simulink model "jMPC_simulinkNL"  (R2022b)
settings: Solver=ode23s  StartTime=0.0  StopTime=simopts.simulink.Tfinal  FixedStep=simopts.Ts  RelTol=1e-3  EnableMultiTasking=on
undefined symbols (not defined in the file): SIMJMPC, simopts
libraries: jMPClib x2, simulink x1
settings Model: Creator=Jonathan  LastModifiedBy=Jonathan Currie
settings SolverCC: AlgebraicLoopSolver=TrustRegion
settings DataIOCC: LimitDataPoints=on  SaveFormat=Array  SignalLoggingSaveFormat=ModelDataLogs  ReturnWorkspaceOutputs=off
settings OptimizationCC: ExpressionDepthLimit=2147483647  LifeSpan=inf
settings DebuggingCC: UnderspecifiedInitializationDetection=Classic  MergeDetectMultiDrivingBlocksExec=none  SolverPrmCheckMsg=warning  FcnCallInpInsideContextMsg=warning  UnconnectedInputMsg=warning  UnconnectedOutputMsg=warning  UnconnectedLineMsg=warning  StateNameClashWarn=warning  SFUnexpectedBacktrackingDiag=warning  SFNoUnconditionalDefaultTransitionDiag=warning  SFExecutionAtInitializationDiag=none  SFMachineParentedDataDiag=warning  ArithmeticOperatorsInVariantConditions=warning
settings HardwareCC: ProdBitPerPointer=32  ProdBitPerSizeT=32  ProdBitPerPtrDiffT=32  ProdLargestAtomicFloat=None  ProdIntDivRoundTo=Undefined  ProdEndianess=Unspecified  ProdWordSize=32  ProdHWDeviceType=32-bit Generic
settings ModelReferenceCC: PropagateSignalLabelsOutOfModel=off
settings SFSimCC: SimUseLocalCustomCode=off  CustomCodeUndefinedFunction=UseInterfaceOnly
settings RTWCC: RTWUseLocalCustomCode=off
settings CodeAppCC: StateflowObjectComments=on
settings GRTTargetCC: TargetLangStandard=C89/C90 (ANSI)  CombineOutputUpdateFcns=off  GRTInterface=on
settings ConfigComp: CovMetricSettings=dw  CovSaveCumulativeToWorkspaceVar=on  CovSaveSingleToWorkspaceVar=on  CovExternalEMLEnable=off

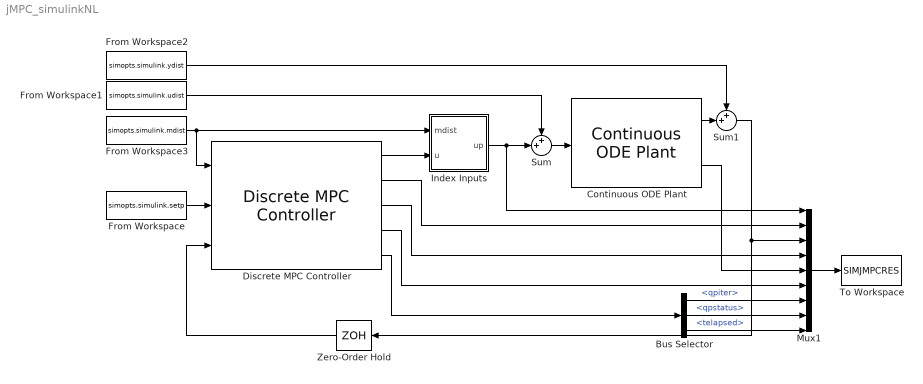
== system jMPC_simulinkNL ==
  Bus Selector : BusSelector  OutputSignals=qpiter,qpstatus,telapsed
  Continuous ODE Plant : jMPClib/MPC Blocks/Continuous ODE Plant  jNLObj=SIMJMPCPlant
      settings: SourceProductName=JMPC Toolbox
  Discrete MPC Controller : jMPClib/MPC Blocks/Discrete MPC Controller  SIMJMPC=SIMJMPC
      settings: SourceProductName=JMPC Toolbox
  From Workspace : FromWorkspace  VariableName=simopts.simulink.setp  SampleTime=simopts.Ts
  From Workspace1 : FromWorkspace  VariableName=simopts.simulink.udist  SampleTime=simopts.Ts
  From Workspace2 : FromWorkspace  VariableName=simopts.simulink.ydist  SampleTime=simopts.Ts
  From Workspace3 : FromWorkspace  VariableName=simopts.simulink.mdist  SampleTime=simopts.Ts
  Index Inputs : Subsystem
  Mux1 : Mux  Inputs=9
  Sum : Sum  Inputs=++|
  Sum1 : Sum  Inputs=++|
  To Workspace : ToWorkspace  VariableName=SIMJMPCRES  SaveFormat=Structure  SampleTime=simopts.Ts
  Zero-Order Hold : ZeroOrderHold  SampleTime=simopts.Ts
  wires:
  Discrete MPC Controller/2 -> Mux1/2
  Mux1/1 -> To Workspace/1
  Sum/1 -> Continuous ODE Plant/1
  Sum1/1 -> Zero-Order Hold/1, Mux1/3
  From Workspace1/1 -> Sum/1
  From Workspace2/1 -> Sum1/1
  Discrete MPC Controller/3 -> Mux1/4
  Discrete MPC Controller/4 -> Mux1/6
  Continuous ODE Plant/1 -> Sum1/2
  Continuous ODE Plant/2 -> Mux1/5
  Zero-Order Hold/1 -> Discrete MPC Controller/3
  From Workspace/1 -> Discrete MPC Controller/2
  Discrete MPC Controller/1 -> Index Inputs/2(u)
  From Workspace3/1 -> Discrete MPC Controller/1, Index Inputs/1(mdist)
  Index Inputs/1(up) -> Sum/2, Mux1/1
  Discrete MPC Controller/5 -> Bus Selector/1
  Bus Selector/1 -> Mux1/7  "<qpiter>"
  Bus Selector/2 -> Mux1/8  "<qpstatus>"
  Bus Selector/3 -> Mux1/9  "<telapsed>"

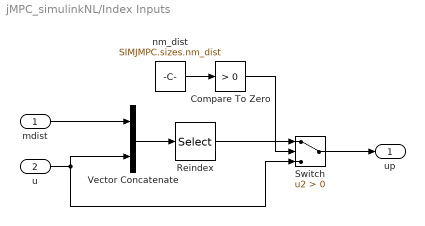
== system jMPC_simulinkNL/Index Inputs ==
  mdist : Inport
  u : Inport  Port=2
  Compare To Zero : simulink/Logic and Bit Operations/Compare To Zero  relop=>  OutDataTypeStr=boolean
  Reindex : Selector  InputPortWidth=SIMJMPC.sizes.nm_in+max(SIMJMPC.sizes.nm_dist,1)  IndexOptions=Index vector (dialog)  Indices=simopts.simulink.mdist_ind  OutputSizes=1
  Switch : Switch  Criteria=u2 > Threshold  SaturateOnIntegerOverflow=off  InputSameDT=off
  Vector Concatenate : Concatenate
  nm_dist : Constant  Value=SIMJMPC.sizes.nm_dist
  up : Outport
  wires:
  u/1 -> Switch/3, Vector Concatenate/2
  Switch/1 -> up/1
  Compare To Zero/1 -> Switch/2
  nm_dist/1 -> Compare To Zero/1
  Vector Concatenate/1 -> Reindex/1
  Reindex/1 -> Switch/1
  mdist/1 -> Vector Concatenate/1
